simulink model "MF52_script"  (R2018b)
settings: Solver=FixedStepAuto  StartTime=0.0  StopTime=10.0  RelTol=1e-3
undefined symbols (not defined in the file or in its folder): mounted_side, par_TIR_front
settings Model: DataDictionary=db_sim_MF52tireparameters.sldd  Creator=ga25xiw  LastModifiedBy=ga25xiw

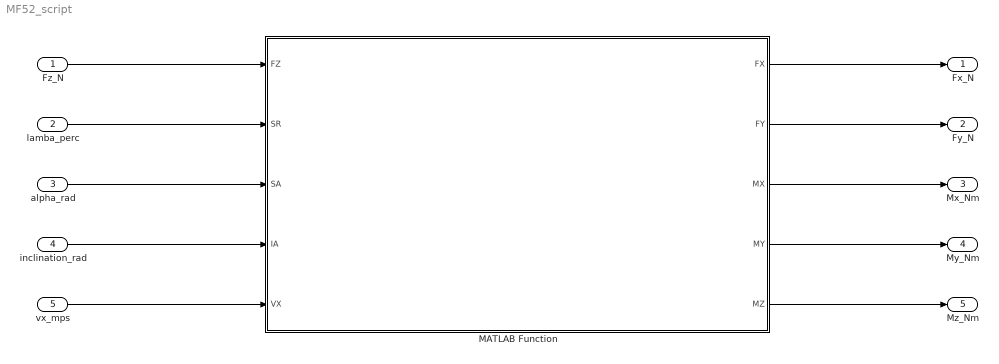
== system MF52_script ==
  Fz_N : Inport
  lamba_perc : Inport  Port=2
  alpha_rad : Inport  Port=3
  inclination_rad : Inport  Port=4
  vx_mps : Inport  Port=5
  MATLAB Function : MATLAB Function  TreatAsAtomicUnit=on
  Fx_N : Outport
  Fy_N : Outport  Port=2
  Mx_Nm : Outport  Port=3
  My_Nm : Outport  Port=4
  Mz_Nm : Outport  Port=5
  wires:
  Fz_N/1 -> MATLAB Function/1(FZ)
  lamba_perc/1 -> MATLAB Function/2(SR)
  alpha_rad/1 -> MATLAB Function/3(SA)
  inclination_rad/1 -> MATLAB Function/4(IA)
  vx_mps/1 -> MATLAB Function/5(VX)
  MATLAB Function/1(FX) -> Fx_N/1
  MATLAB Function/2(FY) -> Fy_N/1
  MATLAB Function/3(MX) -> Mx_Nm/1
  MATLAB Function/4(MY) -> My_Nm/1
  MATLAB Function/5(MZ) -> Mz_Nm/1

== matlab function MF52_script/MATLAB Function ==
  data: FZ input; FX output; SR input; SA input; IA input; VX input; par_TIR_front parameter; mounted_side parameter; FY output; MX output; MY output; MZ output
function [FX, FY, MX, MY, MZ] = MF52_script_wrapper(FZ, SR, SA, IA, VX, par_TIR_front, mounted_side)

    [FX, FY, MX, MY, MZ] = MF_52(FZ, SR, SA, IA, VX, par_TIR_front, mounted_side);
